simulink model "RT_TestMV_ATS"  (R2015b)
settings: Solver=FixedStepDiscrete  StartTime=0.0  StopTime=44.14  FixedStep=samplePeriod  RelTol=1e-3
PreLoadFcn:
  | initialize;
  | scramInitialize;
  | KR_alpha;
  | Discrete_Compensator;
  | ATS_setup
values from neighbouring files (symbols this model uses):
  a_ratio = K2/K1    (= 0.214196975539)    [KR_alpha.m]
  a_sub = ones(DOF_sub,1)    [KR_alpha.m]
  A_sub = (dt*alpha1_sub)/(Msub-Msub*alpha3_sub)    [KR_alpha.m]
  a_sup = ones(DOF_sup,1)    [KR_alpha.m]
  A_sup = (dt*alpha1_sup)/(Msup-Msup*alpha3_sup)    [KR_alpha.m]
  a_vector = ones(DOF,1)    [KR_alpha.m]
  alpha_f_sub = rho_inf_sub/(rho_inf_sub+1)    (= 0.5)    [KR_alpha.m]
  alpha_f_sup = rho_inf_sup/(rho_inf_sup+1)    (= 0.5)    [KR_alpha.m]
  B_sub = ((1/dt)*Msub*alpha3_sub)/alpha1_sub    [KR_alpha.m]
  B_sup = ((1/dt)*Msup*alpha3_sup)/alpha1_sup    [KR_alpha.m]
  controlPeriod = 1/2048    (= 0.00048828125)    [initialize.m]
  Csub = betaKinit*Ksub    [KR_alpha.m]
  Csup = (2*0.01/w1)*Ksup    (= 0.00743030767319)    [KR_alpha.m]
  D_sub = inv(alpha1_sub)/dt    [KR_alpha.m]
  D_sup = inv(alpha1_sup)/dt    [KR_alpha.m]
  dt = samplePeriod    [KR_alpha.m]
  forc_fbk_gain = 1.00    (= 1)    [KR_alpha.m]
  g = 386.089    [KR_alpha.m]
  gamma_sub = 0.5-alpha_m_sub+alpha_f_sub    (= 0.5)    [KR_alpha.m]
  gamma_sup = 0.5-alpha_m_sup+alpha_f_sup    (= 0.5)    [KR_alpha.m]
  K1 = 4.6686*K2    (= 9.3372)    [KR_alpha.m]
  K2 = 0.5*4    (= 2)    [KR_alpha.m]
  Ksub = Kstory    [KR_alpha.m]
  Msub = (0.88585/(56/450))*Mstory    (= 1.03248862309)    [KR_alpha.m]
  Msup = Mstory    (= 0.145044277356)    [KR_alpha.m]
  nAct = 4    [initialize.m]
  nDout = 4    [initialize.m]
  onesec = ceil(1/samplePeriod)    [Discrete_Compensator.m]
  samplePeriod = controlPeriod/upsampleFactor    (= 0.00048828125)    [initialize.m]
  scale_GM = 1.50    (= 1.5)    [KR_alpha.m]
  uy = 0.85    [KR_alpha.m]
undefined symbols (not defined in the file or in its folder): lhpNode, MRC, Nl, P_range, sample, SN, stsNode, Threshold, Zden, Znum
undefined symbols (not defined in the file): HybridCtrlParameters, Par
libraries: simulink x34, slrtlib x8, xpcsystranlib x5
(part 1 of 2)
CloseFcn:
  | rtwprivate ssgencode ModelCloseRequest scrnet_receiver
settings Model: SimulationMode=external  ExtModeArmWhenConnect=off  Creator=mvetsch  LastModifiedBy=Analyst-UCSD
settings SolverCC: EnableConcurrentExecution=on
settings DataIOCC: LimitDataPoints=off  SaveFormat=Array  SignalLoggingSaveFormat=ModelDataLogs  SignalLoggingName=sigsOut
settings OptimizationCC: BlockReduction=off  BooleanDataType=off  OptimizeBlockIOStorage=off  BufferReuse=off  GlobalBufferReuse=off  ExpressionFolding=off  ExpressionDepthLimit=2147483647  LocalBlockOutputs=off  InitFltsAndDblsToZero=on
settings DebuggingCC: SaveWithParameterizedLinksMsg=none  UnderspecifiedInitializationDetection=Classic  MergeDetectMultiDrivingBlocksExec=none  SignalResolutionControl=TryResolveAllWithWarning  MultiTaskDSMMsg=warning  MultiTaskCondExecSysMsg=none  FcnCallInpInsideContextMsg=UseLocalSettings  StateNameClashWarn=warning
settings HardwareCC: ProdBitPerPointer=32  ProdLargestAtomicFloat=None  ProdWordSize=32  ProdLongLongMode=on  ProdHWDeviceType=Generic->32-bit x86 compatible
settings RTWCC: SystemTargetFile=slrt.tlc  TemplateMakefile=slrt_default_tmf  Description=Simulink Real-Time  RTWCompilerOptimization=on
settings SimulinkRealTimeCC: TargetFcnLib=ansi_tfl_tmw.mat  RL32LogBufSizeModifier=10000000  RL32IRQSourceModifier=Auto (PCI only)  xPCIRQSourceBoard=Scramnet_SC150+
settings ConfigComp: CovModelRefEnable=Off

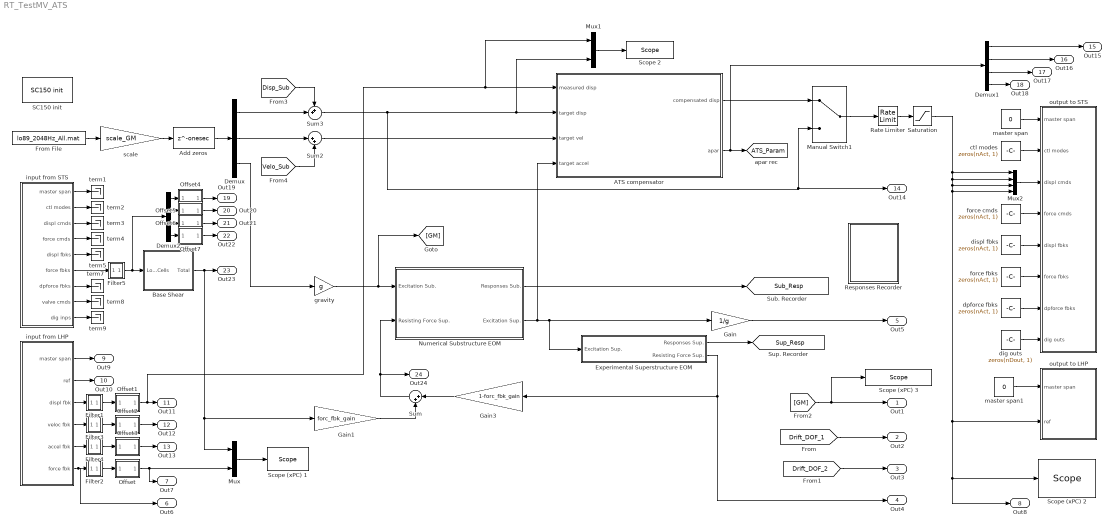
== system RT_TestMV_ATS ==
  ATS compensator : Subsystem  mask{param=Par}
      mask prompts: param "Initial a0, a1, a2 values :"
  Add zeros : Delay  DelayLength=onesec  InitialCondition=0
  Base Shear : Subsystem
  Demux : Demux  Outputs=3
  Demux1 : Demux
  Demux2 : Demux
  Experimental Superstructure EOM : Subsystem
  Filter1 : Subsystem
  Filter2 : Subsystem
  Filter3 : Subsystem
  Filter4 : Subsystem
  Filter5 : Subsystem
  From File : FromFile  FileName=lo89_2048Hz_All.mat  SampleTime=samplePeriod
  Gain : Gain  Gain=1/g
  Gain1 : Gain  Gain=forc_fbk_gain
  Gain3 : Gain  Gain=1-forc_fbk_gain
  Manual Switch1 : ManualSwitch
  Mux : Mux  Inputs=2
  Mux1 : Mux  Inputs=2
  Mux2 : Mux
  Numerical Substructure EOM : Subsystem
  Offset : Subsystem  mask(Signal Offset){nS=HybridCtrlParameters.nDOF, nOffset=onesec}
      mask prompts: nS "Number of Signals: nS"; nOffset "Number of samples to initialize offset: nOffset"
      mask help:
      | Offset signal by average of signal over initial number of samples.
      | Set nOffset = -1 for no signal offset.
      mask Display: fprintf('Signal\nOffset')
  Offset1 : Subsystem  mask(Signal Offset){nS=HybridCtrlParameters.nDOF, nOffset=onesec}
      mask prompts: nS "Number of Signals: nS"; nOffset "Number of samples to initialize offset: nOffset"
      mask help:
      | Offset signal by average of signal over initial number of samples.
      | Set nOffset = -1 for no signal offset.
      mask Display: fprintf('Signal\nOffset')
  Offset2 : Subsystem  mask(Signal Offset){nS=HybridCtrlParameters.nDOF, nOffset=onesec}
      mask prompts: nS "Number of Signals: nS"; nOffset "Number of samples to initialize offset: nOffset"
      mask help:
      | Offset signal by average of signal over initial number of samples.
      | Set nOffset = -1 for no signal offset.
      mask Display: fprintf('Signal\nOffset')
  Offset3 : Subsystem  mask(Signal Offset){nS=HybridCtrlParameters.nDOF, nOffset=onesec}
      mask prompts: nS "Number of Signals: nS"; nOffset "Number of samples to initialize offset: nOffset"
      mask help:
      | Offset signal by average of signal over initial number of samples.
      | Set nOffset = -1 for no signal offset.
      mask Display: fprintf('Signal\nOffset')
  Offset4 : Subsystem  mask(Signal Offset){nS=HybridCtrlParameters.nDOF, nOffset=onesec}
      mask prompts: nS "Number of Signals: nS"; nOffset "Number of samples to initialize offset: nOffset"
      mask help:
      | Offset signal by average of signal over initial number of samples.
      | Set nOffset = -1 for no signal offset.
      mask Display: fprintf('Signal\nOffset')
  Offset5 : Subsystem  mask(Signal Offset){nS=HybridCtrlParameters.nDOF, nOffset=onesec}
      mask prompts: nS "Number of Signals: nS"; nOffset "Number of samples to initialize offset: nOffset"
      mask help:
      | Offset signal by average of signal over initial number of samples.
      | Set nOffset = -1 for no signal offset.
      mask Display: fprintf('Signal\nOffset')
  Offset6 : Subsystem  mask(Signal Offset){nS=HybridCtrlParameters.nDOF, nOffset=onesec}
      mask prompts: nS "Number of Signals: nS"; nOffset "Number of samples to initialize offset: nOffset"
      mask help:
      | Offset signal by average of signal over initial number of samples.
      | Set nOffset = -1 for no signal offset.
      mask Display: fprintf('Signal\nOffset')
  Offset7 : Subsystem  mask(Signal Offset){nS=HybridCtrlParameters.nDOF, nOffset=onesec}
      mask prompts: nS "Number of Signals: nS"; nOffset "Number of samples to initialize offset: nOffset"
      mask help:
      | Offset signal by average of signal over initial number of samples.
      | Set nOffset = -1 for no signal offset.
      mask Display: fprintf('Signal\nOffset')
  Rate Limiter : RateLimiter  RisingSlewLimit=25  FallingSlewLimit=-25  SampleTimeMode=inherited
  Responses Recorder : Subsystem
  SC150 init : xpcsystranlib/Shared Memory/SC150 init   node=node  pci=-1
  Saturation : Saturate  UpperLimit=4.5  LowerLimit=-4.5
  Scope (xPC) 1 : slrtlib/Displays and Logging/Scope   scopeno=2  scopetype=Target  autostart=on  viewmode=Graphical redraw  formatstr='%15.6f'  grid=on  ylimits=[0,0]  nosamples=1024  noprepostsamples=0  interleave=1  triggermode=FreeRun  triggersignal=1  trigsignalfromport=off  triggerlevel=0.0  triggerslope=Either  triggerscope=1  triggersample=0  filename=data.dat  mode=Lazy  writesize=512  autorestart=off  dynamicfilemode=off  maxwritefilesize=512*1024^2
  Scope (xPC) 2 : slrtlib/Displays and Logging/Scope   scopeno=3  scopetype=Target  autostart=on  viewmode=Graphical redraw  formatstr='%15.6f'  grid=on  ylimits=[0,0]  nosamples=1024  noprepostsamples=0  interleave=1  triggermode=FreeRun  triggersignal=1  trigsignalfromport=off  triggerlevel=0.0  triggerslope=Either  triggerscope=1  triggersample=0  filename=data.dat  mode=Lazy  writesize=512  autorestart=off  dynamicfilemode=off  maxwritefilesize=512*1024^2
  Scope (xPC) 3 : slrtlib/Displays and Logging/Scope   scopeno=4  scopetype=Target  autostart=on  viewmode=Graphical redraw  formatstr='%15.6f'  grid=on  ylimits=[0,0]  nosamples=1024  noprepostsamples=0  interleave=1  triggermode=FreeRun  triggersignal=1  trigsignalfromport=off  triggerlevel=0.0  triggerslope=Either  triggerscope=1  triggersample=0  filename=data.dat  mode=Lazy  writesize=512  autorestart=off  dynamicfilemode=off  maxwritefilesize=512*1024^2
  Scope 2 : slrtlib/Displays and Logging/Scope   scopeno=1  scopetype=Target  autostart=on  viewmode=Graphical redraw  formatstr='%15.6f'  grid=on  ylimits=[0,0]  nosamples=250  noprepostsamples=0  interleave=1  triggermode=FreeRun  triggersignal=1  trigsignalfromport=off  triggerlevel=0.0  triggerslope=Either  triggerscope=1  triggersample=0  filename=data.dat  mode=Lazy  writesize=512  autorestart=off  dynamicfilemode=off  maxwritefilesize=512*1024^2
  Sum : Sum  Inputs=|++
  Sum2 : Sum  Inputs=|++
  Sum3 : Sum  Inputs=++|
  ctl modes : Constant  Value=zeros(nAct, 1)
  dig outs : Constant  Value=zeros(nDout, 1)  OutDataTypeStr=uint32
  displ fbks : Constant  Value=zeros(nAct, 1)
  dpforce fbks : Constant  Value=zeros(nAct, 1)
  force cmds : Constant  Value=zeros(nAct, 1)
  force fbks : Constant  Value=zeros(nAct, 1)
  gravity : Gain  Gain=g
  input from LHP : Subsystem
  input from STS : Subsystem
  master span : Constant  Value=0
  master span1 : Constant  Value=0
  output to LHP : Subsystem
  output to STS : Subsystem
  scale : Gain  Gain=scale_GM
  term{1..5,7..9} (8 alike) : Terminator
  Out1 : Outport  SampleTime=samplePeriod
  Out2 : Outport  Port=2  SampleTime=samplePeriod
  Out3 : Outport  Port=3  SampleTime=samplePeriod
  Out4 : Outport  Port=4  SampleTime=samplePeriod
  Out5 : Outport  Port=5  SampleTime=samplePeriod
  Out6 : Outport  Port=6  SampleTime=samplePeriod
  Out7 : Outport  Port=7  SampleTime=samplePeriod
  Out8 : Outport  Port=8  SampleTime=samplePeriod
  Out9 : Outport  Port=9  SampleTime=samplePeriod
  Out10 : Outport  Port=10  SampleTime=samplePeriod
  Out11 : Outport  Port=11  SampleTime=samplePeriod
  Out12 : Outport  Port=12  SampleTime=samplePeriod
  Out13 : Outport  Port=13  SampleTime=samplePeriod
  Out14 : Outport  Port=14
  Out15 : Outport  Port=15
  Out16 : Outport  Port=16
  Out17 : Outport  Port=17
  Out18 : Outport  Port=18
  Out19 : Outport  Port=19
  Out20 : Outport  Port=20
  Out21 : Outport  Port=21
  Out22 : Outport  Port=22
  Out23 : Outport  Port=23
  Out24 : Outport  Port=24
  tag scope: ATS_Param=global, Sub_Resp=global, Sup_Resp=global
  wires:
  master span/1 -> output to STS/1(master span)
  ctl modes/1 -> output to STS/2(ctl modes)
  force cmds/1 -> output to STS/4(force cmds)
  displ fbks/1 -> output to STS/5(displ fbks)
  force fbks/1 -> output to STS/6(force fbks)
  dpforce fbks/1 -> output to STS/7(dpforce fbks)
  input from STS/4(force cmds) -> term4/1
  input from STS/5(displ fbks) -> term5/1
  input from STS/6(force fbks) -> Filter5/1(In1)
  input from STS/7(dpforce fbks) -> term7/1
  input from STS/8(valve cmds) -> term8/1
  input from STS/9(dig inps) -> term9/1
  dig outs/1 -> output to STS/8(dig outs)
  input from LHP/1(master span) -> Out9/1
  input from LHP/3(displ fbk) -> Filter1/1(In1)
  input from LHP/4(veloc fbk) -> Filter3/1(In1)
  input from LHP/5(accel fbk) -> Filter4/1(In1)
  Mux/1 -> Scope (xPC) 1/1
  input from LHP/6(force fbk) -> Out6/1, Filter2/1(In1)
  Numerical Substructure EOM/1(Responses Sub.) -> [Sub_Resp]
  Experimental Superstructure EOM/1(Responses Sup.) -> [Sup_Resp]
  [Drift_DOF_1] -> Out2/1
  [Drift_DOF_2] -> Out3/1
  master span1/1 -> output to LHP/1(master span)
  Filter2/1(Out1) -> Offset/1(In1)
  Offset/1(Out1) -> Out7/1, Mux/2
  input from LHP/2(ref) -> Out10/1
  From File/1 -> scale/1
  gravity/1 -> [GM], Numerical Substructure EOM/1(Excitation Sub.)
  Sum/1 -> Out24/1, Numerical Substructure EOM/2(Resisting Force Sup.)
  Experimental Superstructure EOM/2(Resisting Force Sup.) -> Out4/1, Gain3/1
  [GM] -> Scope (xPC) 3/1, Out1/1
  Numerical Substructure EOM/2(Excitation Sup.) -> Gain/1, Experimental Superstructure EOM/1(Excitation Sup.), ATS compensator/4(target accel)
  Gain1/1 -> Sum/2
  Add zeros/1 -> Demux/1
  Demux/3 -> gravity/1
  [Disp_Sub] -> Sum3/1
  Gain/1 -> Out5/1
  scale/1 -> Add zeros/1
  input from STS/1(master span) -> term1/1
  Sum3/1 -> Mux1/2, ATS compensator/2(target disp), Manual Switch1/2, Out14/1
  Sum2/1 -> ATS compensator/3(target vel)
  Manual Switch1/1 -> Rate Limiter/1
  ATS compensator/1(compensated disp) -> Manual Switch1/1
  ATS compensator/2(apar) -> [ATS_Param], Demux1/1
  Rate Limiter/1 -> Saturation/1
  Saturation/1 -> Mux2/1, Mux2/2, Mux2/3, Mux2/4, Scope (xPC) 2/1, Out8/1, output to LHP/2(ref)
  Demux1/1 -> Out15/1
  Demux1/2 -> Out16/1
  Demux1/3 -> Out17/1
  Demux1/4 -> Out18/1
  Offset1/1(Out1) -> Mux1/1, ATS compensator/1(measured disp), Out11/1
  Gain3/1 -> Sum/1
  Filter1/1(Out1) -> Offset1/1(In1)
  Mux2/1 -> output to STS/3(displ cmds)
  input from STS/2(ctl modes) -> term2/1
  input from STS/3(displ cmds) -> term3/1
  Demux2/1 -> Offset4/1(In1)
  Demux2/2 -> Offset5/1(In1)
  Demux2/3 -> Offset6/1(In1)
  Demux2/4 -> Offset7/1(In1)
  Base Shear/1(Total) -> Mux/1, Gain1/1, Out23/1
  Filter3/1(Out1) -> Offset2/1(In1)
  Filter4/1(Out1) -> Offset3/1(In1)
  Offset2/1(Out1) -> Out12/1
  Offset3/1(Out1) -> Out13/1
  Filter5/1(Out1) -> Base Shear/1(Load Cells), Demux2/1
  Offset4/1(Out1) -> Out19/1
  Offset5/1(Out1) -> Out20/1
  Offset6/1(Out1) -> Out21/1
  Offset7/1(Out1) -> Out22/1
  Mux1/1 -> Scope 2/1
  Demux/2 -> Sum2/1
  [Velo_Sub] -> Sum2/2
  Demux/1 -> Sum3/2

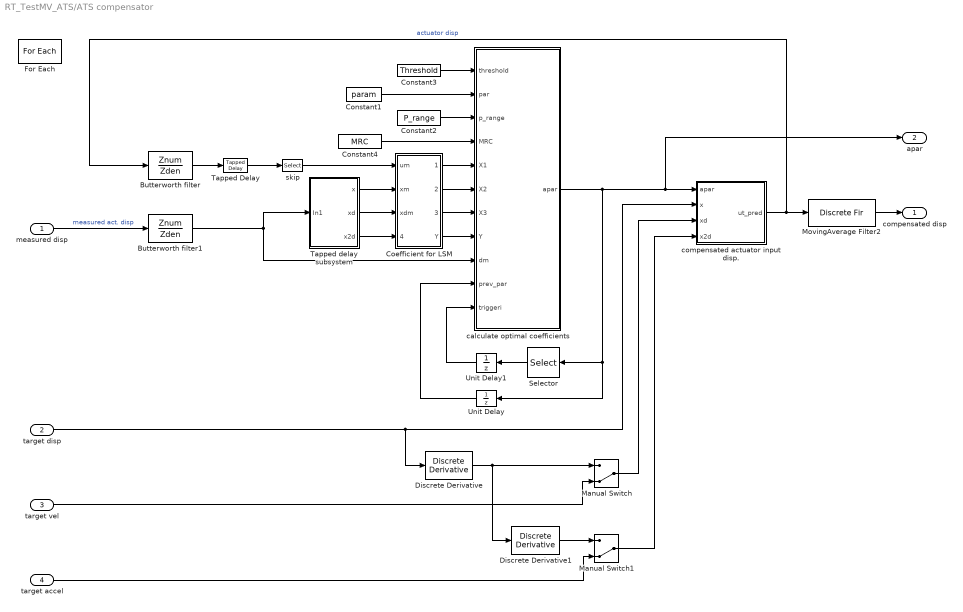
== system RT_TestMV_ATS/ATS compensator ==
  measured disp : Inport  Partition=on  PartitionDimension=1  PartitionWidth=1
  target disp : Inport  Port=2  Partition=on  PartitionDimension=1  PartitionWidth=1
  target vel : Inport  Port=3  Partition=on  PartitionDimension=1  PartitionWidth=1
  target accel : Inport  Port=4  Partition=on  PartitionDimension=1  PartitionWidth=1
  Butterworth filter : DiscreteTransferFcn  Numerator=Znum  Denominator=Zden  SampleTime=sample
  Butterworth filter1 : DiscreteTransferFcn  Numerator=Znum  Denominator=Zden  SampleTime=sample
  Coefficient for LSM : Subsystem
  Constant1 : Constant  Value=param
  Constant2 : Constant  Value=P_range
  Constant3 : Constant  Value=Threshold
  Constant4 : Constant  Value=MRC
  Discrete Derivative : simulink/Discrete/Discrete Derivative  gainval=1.0  ICPrevScaledInput=0.0  OutMin=[]  OutMax=[]  OutDataType=fixdt(1, 16)  OutScaling=2^-10  DoSatur=off
  Discrete Derivative1 : simulink/Discrete/Discrete Derivative  gainval=1.0  ICPrevScaledInput=0.0  OutMin=[]  OutMax=[]  OutDataType=fixdt(1, 16)  OutScaling=2^-10  DoSatur=off
  For Each : ForEach  DisableCoverage=on  IterateSubsysMaskParameter=on  SubsysMaskParameterIterationDimension=2  IndexMode=One-based
  Manual Switch : ManualSwitch  CurrentSetting=0
  Manual Switch1 : ManualSwitch  CurrentSetting=0
  MovingAverage Filter2 : DiscreteFir  Coefficients=1/numSample*ones(1,numSample)  mask(Moving Average Filter){numSample=10}
      mask prompts: numSample "Number of Samples: numSample"
      mask help:
      | Moving average filter by using discrete FIR filter.
      | Set numSample = 1 for no filtering.
      mask Display: fprintf('MovingAverage\nFilter')
  Selector : Selector  InputPortWidth=4  IndexOptions=Index vector (dialog)  Indices=4  OutputSizes=1
  Tapped Delay : simulink/Discrete/Tapped Delay  vinit=0.0  samptime=-1  NumDelays=Nl  DelayOrder=Oldest  includeCurrent=off
  Tapped delay subsystem : Subsystem
  Unit Delay : UnitDelay  SampleTime=-1
  Unit Delay1 : UnitDelay  SampleTime=-1
  calculate optimal coefficients : MATLAB Function  TreatAsAtomicUnit=on
  compensated actuator input disp. : MATLAB Function  TreatAsAtomicUnit=on
  skip : Selector  InputPortWidth=Nl  IndexOptions=Index vector (dialog)  Indices=[1:SN:Nl]  OutputSizes=1
  compensated disp : Outport  ConcatenationDimension=1
  apar : Outport  Port=2  ConcatenationDimension=1
  wires:
  measured disp/1 -> Butterworth filter1/1  "measured act. disp"
  Tapped Delay/1 -> skip/1
  calculate optimal coefficients/1(apar) -> Unit Delay/1, Selector/1, apar/1, compensated actuator input disp./1(apar)
  compensated actuator input disp./1(ut_pred) -> Butterworth filter/1, MovingAverage Filter2/1  "actuator disp"
  Constant1/1 -> calculate optimal coefficients/2(par)
  Constant2/1 -> calculate optimal coefficients/3(p_range)
  Unit Delay/1 -> calculate optimal coefficients/10(prev_par)
  target disp/1 -> compensated actuator input disp./2(x), Discrete Derivative/1
  skip/1 -> Coefficient for LSM/1(um)
  Tapped delay subsystem/1(x) -> Coefficient for LSM/2(xm)
  Tapped delay subsystem/2(xd) -> Coefficient for LSM/3(xdm)
  Tapped delay subsystem/3(x2d) -> Coefficient for LSM/4(x2dm)
  Coefficient for LSM/1(X(1,:)) -> calculate optimal coefficients/5(X1)
  Coefficient for LSM/2(X(2,:)) -> calculate optimal coefficients/6(X2)
  Coefficient for LSM/3(X(3,:)) -> calculate optimal coefficients/7(X3)
  Coefficient for LSM/4(Y) -> calculate optimal coefficients/8(Y)
  Unit Delay1/1 -> calculate optimal coefficients/11(triggeri)
  Constant3/1 -> calculate optimal coefficients/1(threshold)
  Butterworth filter/1 -> Tapped Delay/1
  Constant4/1 -> calculate optimal coefficients/4(MRC)
  Selector/1 -> Unit Delay1/1
  Manual Switch/1 -> compensated actuator input disp./3(xd)
  Discrete Derivative/1 -> Manual Switch/1, Discrete Derivative1/1
  target vel/1 -> Manual Switch/2
  Discrete Derivative1/1 -> Manual Switch1/1
  Manual Switch1/1 -> compensated actuator input disp./4(x2d)
  target accel/1 -> Manual Switch1/2
  Butterworth filter1/1 -> Tapped delay subsystem/1(In1), calculate optimal coefficients/9(dm)
  MovingAverage Filter2/1 -> compensated disp/1

== system RT_TestMV_ATS/Base Shear ==
  Load Cells : Inport
  Demux : Demux
  Offset1 : Subsystem  mask(Signal Offset){nS=HybridCtrlParameters.nDOF, nOffset=onesec}
      mask prompts: nS "Number of Signals: nS"; nOffset "Number of samples to initialize offset: nOffset"
      mask help:
      | Offset signal by average of signal over initial number of samples.
      | Set nOffset = -1 for no signal offset.
      mask Display: fprintf('Signal\nOffset')
  Offset2 : Subsystem  mask(Signal Offset){nS=HybridCtrlParameters.nDOF, nOffset=onesec}
      mask prompts: nS "Number of Signals: nS"; nOffset "Number of samples to initialize offset: nOffset"
      mask help:
      | Offset signal by average of signal over initial number of samples.
      | Set nOffset = -1 for no signal offset.
      mask Display: fprintf('Signal\nOffset')
  Offset3 : Subsystem  mask(Signal Offset){nS=HybridCtrlParameters.nDOF, nOffset=onesec}
      mask prompts: nS "Number of Signals: nS"; nOffset "Number of samples to initialize offset: nOffset"
      mask help:
      | Offset signal by average of signal over initial number of samples.
      | Set nOffset = -1 for no signal offset.
      mask Display: fprintf('Signal\nOffset')
  Offset4 : Subsystem  mask(Signal Offset){nS=HybridCtrlParameters.nDOF, nOffset=onesec}
      mask prompts: nS "Number of Signals: nS"; nOffset "Number of samples to initialize offset: nOffset"
      mask help:
      | Offset signal by average of signal over initial number of samples.
      | Set nOffset = -1 for no signal offset.
      mask Display: fprintf('Signal\nOffset')
  Sum : Sum  Inputs=++++
  Total : Outport
  wires:
  Demux/3 -> Offset2/1(In1)
  Demux/4 -> Offset3/1(In1)
  Demux/2 -> Offset1/1(In1)
  Demux/1 -> Offset4/1(In1)
  Load Cells/1 -> Demux/1
  Sum/1 -> Total/1
  Offset4/1(Out1) -> Sum/1
  Offset1/1(Out1) -> Sum/2
  Offset2/1(Out1) -> Sum/3
  Offset3/1(Out1) -> Sum/4

== system RT_TestMV_ATS/Experimental Superstructure EOM ==
  Excitation Sup. : Inport
  Delay1 : Delay  DelayLength=1
  Demux : Demux  Outputs=3
  Demux1 : Demux  Outputs=3
  Gain : Gain  Gain=Csup  Multiplication=Matrix(K*u) (u vector)
  Gain2 : Gain  Gain=-Msup*a_sup  Multiplication=Matrix(K*u)
  Material : Subsystem
  Subsystem : Subsystem
  Sum : Sum  Inputs=|++
  Terminator{,1..3} (4 alike) : Terminator
  Responses Sup. : Outport
  Resisting Force Sup. : Outport  Port=2
  wires:
  Subsystem/1(Responses i+1) -> Demux1/1, Demux/1, Delay1/1, Responses Sup./1
  Excitation Sup./1 -> Gain2/1
  Demux1/2 -> Gain/1
  Sum/1 -> Resisting Force Sup./1
  Demux/1 -> Material/1(Disp)
  Demux/3 -> Terminator/1
  Demux/2 -> Terminator1/1
  Demux1/1 -> Terminator2/1
  Demux1/3 -> Terminator3/1
  Gain/1 -> Sum/1
  Delay1/1 -> Subsystem/3(Responses i)
  Material/1(Force) -> Sum/2, Subsystem/2(Restoring A/E)
  Gain2/1 -> Subsystem/1(Excitation Force)

== system RT_TestMV_ATS/Filter1 ==
  In1 : Inport
  MovingAverage Filter2 : DiscreteFir  Coefficients=1/numSample*ones(1,numSample)  mask(Moving Average Filter){numSample=7}
      mask prompts: numSample "Number of Samples: numSample"
      mask help:
      | Moving average filter by using discrete FIR filter.
      | Set numSample = 1 for no filtering.
      mask Display: fprintf('MovingAverage\nFilter')
  Out1 : Outport
  wires:
  In1/1 -> MovingAverage Filter2/1
  MovingAverage Filter2/1 -> Out1/1

== system RT_TestMV_ATS/Filter2 ==
  In1 : Inport
  MovingAverage Filter2 : DiscreteFir  Coefficients=1/numSample*ones(1,numSample)  mask(Moving Average Filter){numSample=7}
      mask prompts: numSample "Number of Samples: numSample"
      mask help:
      | Moving average filter by using discrete FIR filter.
      | Set numSample = 1 for no filtering.
      mask Display: fprintf('MovingAverage\nFilter')
  Out1 : Outport
  wires:
  In1/1 -> MovingAverage Filter2/1
  MovingAverage Filter2/1 -> Out1/1

== system RT_TestMV_ATS/Filter3 ==
  In1 : Inport
  MovingAverage Filter2 : DiscreteFir  Coefficients=1/numSample*ones(1,numSample)  mask(Moving Average Filter){numSample=7}
      mask prompts: numSample "Number of Samples: numSample"
      mask help:
      | Moving average filter by using discrete FIR filter.
      | Set numSample = 1 for no filtering.
      mask Display: fprintf('MovingAverage\nFilter')
  Out1 : Outport
  wires:
  In1/1 -> MovingAverage Filter2/1
  MovingAverage Filter2/1 -> Out1/1

== system RT_TestMV_ATS/Filter4 ==
  In1 : Inport
  MovingAverage Filter2 : DiscreteFir  Coefficients=1/numSample*ones(1,numSample)  mask(Moving Average Filter){numSample=7}
      mask prompts: numSample "Number of Samples: numSample"
      mask help:
      | Moving average filter by using discrete FIR filter.
      | Set numSample = 1 for no filtering.
      mask Display: fprintf('MovingAverage\nFilter')
  Out1 : Outport
  wires:
  In1/1 -> MovingAverage Filter2/1
  MovingAverage Filter2/1 -> Out1/1

== system RT_TestMV_ATS/Filter5 ==
  In1 : Inport
  MovingAverage Filter2 : DiscreteFir  Coefficients=1/numSample*ones(1,numSample)  mask(Moving Average Filter){numSample=7}
      mask prompts: numSample "Number of Samples: numSample"
      mask help:
      | Moving average filter by using discrete FIR filter.
      | Set numSample = 1 for no filtering.
      mask Display: fprintf('MovingAverage\nFilter')
  Out1 : Outport
  wires:
  In1/1 -> MovingAverage Filter2/1
  MovingAverage Filter2/1 -> Out1/1

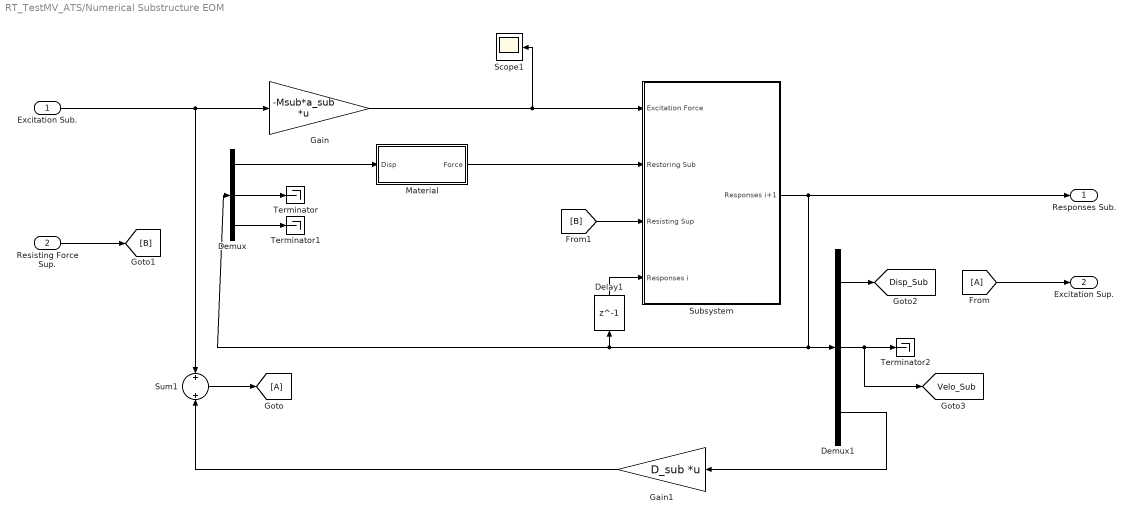
== system RT_TestMV_ATS/Numerical Substructure EOM ==
  Excitation Sub. : Inport
  Resisting Force Sup. : Inport  Port=2
  Delay1 : Delay  DelayLength=1
  Demux : Demux  Outputs=3
  Demux1 : Demux  Outputs=3
  Gain : Gain  Gain=-Msub*a_sub  Multiplication=Matrix(K*u)
  Gain1 : Gain  Gain=D_sub  Multiplication=Matrix(K*u) (u vector)
  Material : Subsystem
  Scope1 : Scope
  Subsystem : Subsystem
  Sum1 : Sum  Inputs=+||+
  Terminator : Terminator
  Terminator1 : Terminator
  Terminator2 : Terminator
  Responses Sub. : Outport
  Excitation Sup. : Outport  Port=2
  tag scope: Disp_Sub=global, Velo_Sub=global
  wires:
  Gain/1 -> Scope1/1, Subsystem/1(Excitation Force)
  Subsystem/1(Responses i+1) -> Demux/1, Delay1/1, Demux1/1, Responses Sub./1
  Demux/1 -> Material/1(Disp)
  Excitation Sub./1 -> Sum1/1, Gain/1
  Demux1/3 -> Gain1/1
  Demux/2 -> Terminator/1
  Demux/3 -> Terminator1/1
  Demux1/1 -> [Disp_Sub]
  Delay1/1 -> Subsystem/4(Responses i)
  Material/1(Force) -> Subsystem/2(Restoring Sub)
  Gain1/1 -> Sum1/2
  Demux1/2 -> [Velo_Sub], Terminator2/1
  Sum1/1 -> [A]
  [A] -> Excitation Sup./1
  Resisting Force Sup./1 -> [B]
  [B] -> Subsystem/3(Resisting Sup)

== system RT_TestMV_ATS/Offset ==
  In1 : Inport
  Constant : Constant  Value=zeros(1,nS)
  Counter : simulink/Sources/Counter Free-Running  NumBits=32  tsamp=-1
  Data Store Memory : DataStoreMemory  DataStoreName=x0  InitialValue=zeros(1,nS)  OutDataTypeStr=double
  Data Store Read : DataStoreRead  DataStoreName=x0  SampleTime=controlPeriod
  If : If  IfExpression=u1 < nOffset  ShowElse=off
  If Action : Subsystem  TreatAsAtomicUnit=on
  Sum1 : Sum  Inputs=+-|  SaturateOnIntegerOverflow=on  InputSameDT=on  OutDataTypeStr=Inherit: Same as first input
  Switch : Switch  Threshold=nOffset  SaturateOnIntegerOverflow=on  InputSameDT=on
  typeConv2 : DataTypeConversion  OutDataTypeStr=double  SaturateOnIntegerOverflow=on  RndMeth=Zero
  Out1 : Outport
  wires:
  Switch/1 -> Out1/1
  Sum1/1 -> Switch/1
  Data Store Read/1 -> Sum1/2
  In1/1 -> If Action/1(In1), Sum1/1
  Constant/1 -> Switch/3
  Counter/1 -> typeConv2/1
  If/1 -> If Action/Action
  typeConv2/1 -> Switch/2, If/1

== system RT_TestMV_ATS/Offset1 ==
  In1 : Inport
  Constant : Constant  Value=zeros(1,nS)
  Counter : simulink/Sources/Counter Free-Running  NumBits=32  tsamp=-1
  Data Store Memory : DataStoreMemory  DataStoreName=x0  InitialValue=zeros(1,nS)  OutDataTypeStr=double
  Data Store Read : DataStoreRead  DataStoreName=x0  SampleTime=controlPeriod
  If : If  IfExpression=u1 < nOffset  ShowElse=off
  If Action : Subsystem  TreatAsAtomicUnit=on
  Sum1 : Sum  Inputs=+-|  SaturateOnIntegerOverflow=on  InputSameDT=on  OutDataTypeStr=Inherit: Same as first input
  Switch : Switch  Threshold=nOffset  SaturateOnIntegerOverflow=on  InputSameDT=on
  typeConv2 : DataTypeConversion  OutDataTypeStr=double  SaturateOnIntegerOverflow=on  RndMeth=Zero
  Out1 : Outport
  wires:
  Switch/1 -> Out1/1
  Sum1/1 -> Switch/1
  Data Store Read/1 -> Sum1/2
  In1/1 -> If Action/1(In1), Sum1/1
  Constant/1 -> Switch/3
  Counter/1 -> typeConv2/1
  If/1 -> If Action/Action
  typeConv2/1 -> Switch/2, If/1

== system RT_TestMV_ATS/Offset2 ==
  In1 : Inport
  Constant : Constant  Value=zeros(1,nS)
  Counter : simulink/Sources/Counter Free-Running  NumBits=32  tsamp=-1
  Data Store Memory : DataStoreMemory  DataStoreName=x0  InitialValue=zeros(1,nS)  OutDataTypeStr=double
  Data Store Read : DataStoreRead  DataStoreName=x0  SampleTime=controlPeriod
  If : If  IfExpression=u1 < nOffset  ShowElse=off
  If Action : Subsystem  TreatAsAtomicUnit=on
  Sum1 : Sum  Inputs=+-|  SaturateOnIntegerOverflow=on  InputSameDT=on  OutDataTypeStr=Inherit: Same as first input
  Switch : Switch  Threshold=nOffset  SaturateOnIntegerOverflow=on  InputSameDT=on
  typeConv2 : DataTypeConversion  OutDataTypeStr=double  SaturateOnIntegerOverflow=on  RndMeth=Zero
  Out1 : Outport
  wires:
  Switch/1 -> Out1/1
  Sum1/1 -> Switch/1
  Data Store Read/1 -> Sum1/2
  In1/1 -> If Action/1(In1), Sum1/1
  Constant/1 -> Switch/3
  Counter/1 -> typeConv2/1
  If/1 -> If Action/Action
  typeConv2/1 -> Switch/2, If/1

== system RT_TestMV_ATS/Offset3 ==
  In1 : Inport
  Constant : Constant  Value=zeros(1,nS)
  Counter : simulink/Sources/Counter Free-Running  NumBits=32  tsamp=-1
  Data Store Memory : DataStoreMemory  DataStoreName=x0  InitialValue=zeros(1,nS)  OutDataTypeStr=double
  Data Store Read : DataStoreRead  DataStoreName=x0  SampleTime=controlPeriod
  If : If  IfExpression=u1 < nOffset  ShowElse=off
  If Action : Subsystem  TreatAsAtomicUnit=on
  Sum1 : Sum  Inputs=+-|  SaturateOnIntegerOverflow=on  InputSameDT=on  OutDataTypeStr=Inherit: Same as first input
  Switch : Switch  Threshold=nOffset  SaturateOnIntegerOverflow=on  InputSameDT=on
  typeConv2 : DataTypeConversion  OutDataTypeStr=double  SaturateOnIntegerOverflow=on  RndMeth=Zero
  Out1 : Outport
  wires:
  Switch/1 -> Out1/1
  Sum1/1 -> Switch/1
  Data Store Read/1 -> Sum1/2
  In1/1 -> If Action/1(In1), Sum1/1
  Constant/1 -> Switch/3
  Counter/1 -> typeConv2/1
  If/1 -> If Action/Action
  typeConv2/1 -> Switch/2, If/1

== system RT_TestMV_ATS/Offset4 ==
  In1 : Inport
  Constant : Constant  Value=zeros(1,nS)
  Counter : simulink/Sources/Counter Free-Running  NumBits=32  tsamp=-1
  Data Store Memory : DataStoreMemory  DataStoreName=x0  InitialValue=zeros(1,nS)  OutDataTypeStr=double
  Data Store Read : DataStoreRead  DataStoreName=x0  SampleTime=controlPeriod
  If : If  IfExpression=u1 < nOffset  ShowElse=off
  If Action : Subsystem  TreatAsAtomicUnit=on
  Sum1 : Sum  Inputs=+-|  SaturateOnIntegerOverflow=on  InputSameDT=on  OutDataTypeStr=Inherit: Same as first input
  Switch : Switch  Threshold=nOffset  SaturateOnIntegerOverflow=on  InputSameDT=on
  typeConv2 : DataTypeConversion  OutDataTypeStr=double  SaturateOnIntegerOverflow=on  RndMeth=Zero
  Out1 : Outport
  wires:
  Switch/1 -> Out1/1
  Sum1/1 -> Switch/1
  Data Store Read/1 -> Sum1/2
  In1/1 -> If Action/1(In1), Sum1/1
  Constant/1 -> Switch/3
  Counter/1 -> typeConv2/1
  If/1 -> If Action/Action
  typeConv2/1 -> Switch/2, If/1

== system RT_TestMV_ATS/Offset5 ==
  In1 : Inport
  Constant : Constant  Value=zeros(1,nS)
  Counter : simulink/Sources/Counter Free-Running  NumBits=32  tsamp=-1
  Data Store Memory : DataStoreMemory  DataStoreName=x0  InitialValue=zeros(1,nS)  OutDataTypeStr=double
  Data Store Read : DataStoreRead  DataStoreName=x0  SampleTime=controlPeriod
  If : If  IfExpression=u1 < nOffset  ShowElse=off
  If Action : Subsystem  TreatAsAtomicUnit=on
  Sum1 : Sum  Inputs=+-|  SaturateOnIntegerOverflow=on  InputSameDT=on  OutDataTypeStr=Inherit: Same as first input
  Switch : Switch  Threshold=nOffset  SaturateOnIntegerOverflow=on  InputSameDT=on
  typeConv2 : DataTypeConversion  OutDataTypeStr=double  SaturateOnIntegerOverflow=on  RndMeth=Zero
  Out1 : Outport
  wires:
  Switch/1 -> Out1/1
  Sum1/1 -> Switch/1
  Data Store Read/1 -> Sum1/2
  In1/1 -> If Action/1(In1), Sum1/1
  Constant/1 -> Switch/3
  Counter/1 -> typeConv2/1
  If/1 -> If Action/Action
  typeConv2/1 -> Switch/2, If/1

== system RT_TestMV_ATS/Offset6 ==
  In1 : Inport
  Constant : Constant  Value=zeros(1,nS)
  Counter : simulink/Sources/Counter Free-Running  NumBits=32  tsamp=-1
  Data Store Memory : DataStoreMemory  DataStoreName=x0  InitialValue=zeros(1,nS)  OutDataTypeStr=double
  Data Store Read : DataStoreRead  DataStoreName=x0  SampleTime=controlPeriod
  If : If  IfExpression=u1 < nOffset  ShowElse=off
  If Action : Subsystem  TreatAsAtomicUnit=on
  Sum1 : Sum  Inputs=+-|  SaturateOnIntegerOverflow=on  InputSameDT=on  OutDataTypeStr=Inherit: Same as first input
  Switch : Switch  Threshold=nOffset  SaturateOnIntegerOverflow=on  InputSameDT=on
  typeConv2 : DataTypeConversion  OutDataTypeStr=double  SaturateOnIntegerOverflow=on  RndMeth=Zero
  Out1 : Outport
  wires:
  Switch/1 -> Out1/1
  Sum1/1 -> Switch/1
  Data Store Read/1 -> Sum1/2
  In1/1 -> If Action/1(In1), Sum1/1
  Constant/1 -> Switch/3
  Counter/1 -> typeConv2/1
  If/1 -> If Action/Action
  typeConv2/1 -> Switch/2, If/1

== system RT_TestMV_ATS/Offset7 ==
  In1 : Inport
  Constant : Constant  Value=zeros(1,nS)
  Counter : simulink/Sources/Counter Free-Running  NumBits=32  tsamp=-1
  Data Store Memory : DataStoreMemory  DataStoreName=x0  InitialValue=zeros(1,nS)  OutDataTypeStr=double
  Data Store Read : DataStoreRead  DataStoreName=x0  SampleTime=controlPeriod
  If : If  IfExpression=u1 < nOffset  ShowElse=off
  If Action : Subsystem  TreatAsAtomicUnit=on
  Sum1 : Sum  Inputs=+-|  SaturateOnIntegerOverflow=on  InputSameDT=on  OutDataTypeStr=Inherit: Same as first input
  Switch : Switch  Threshold=nOffset  SaturateOnIntegerOverflow=on  InputSameDT=on
  typeConv2 : DataTypeConversion  OutDataTypeStr=double  SaturateOnIntegerOverflow=on  RndMeth=Zero
  Out1 : Outport
  wires:
  Switch/1 -> Out1/1
  Sum1/1 -> Switch/1
  Data Store Read/1 -> Sum1/2
  In1/1 -> If Action/1(In1), Sum1/1
  Constant/1 -> Switch/3
  Counter/1 -> typeConv2/1
  If/1 -> If Action/Action
  typeConv2/1 -> Switch/2, If/1

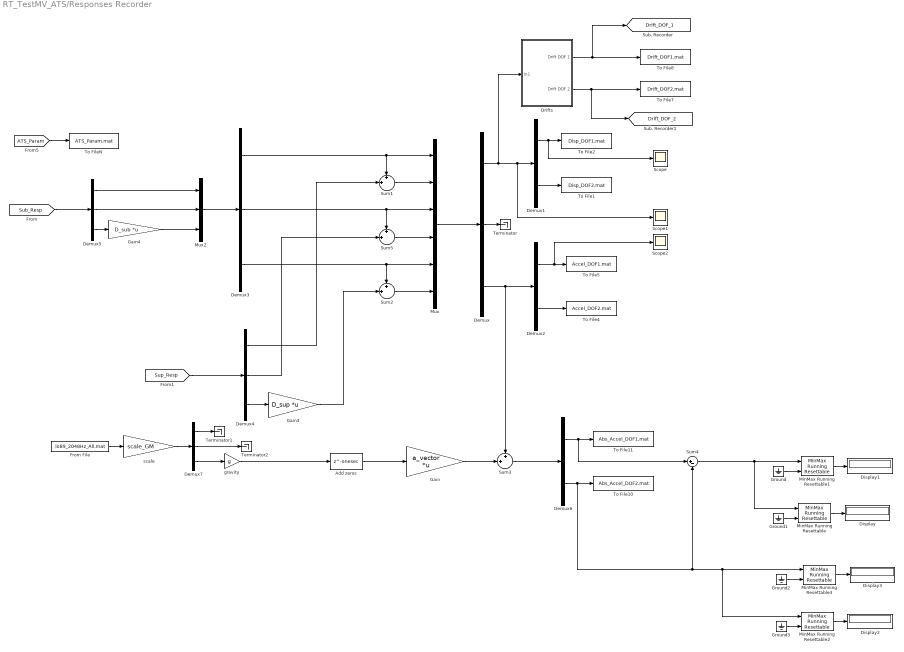
== system RT_TestMV_ATS/Responses Recorder ==
  Add zeros : Delay  DelayLength=onesec  InitialCondition=0
  Demux{,3..5,7} (5 alike) : Demux  Outputs=3
  Demux1 : Demux  Outputs=2
  Demux2 : Demux  Outputs=2
  Demux6 : Demux  Outputs=2
  Display{,1..3} (4 alike) : Display
  Drifts : Subsystem
  From File : FromFile  FileName=lo89_2048Hz_All.mat  SampleTime=samplePeriod
  Gain : Gain  Gain=a_vector  Multiplication=Matrix(K*u)
  Gain3 : Gain  Gain=D_sup  Multiplication=Matrix(K*u) (u vector)
  Gain4 : Gain  Gain=D_sub  Multiplication=Matrix(K*u) (u vector)
  Ground{,1..3} (4 alike) : Ground
  MinMax Running Resettable : simulink/Math Operations/MinMax Running Resettable  Function=max  vinit=0.0
  MinMax Running Resettable1 : simulink/Math Operations/MinMax Running Resettable  Function=min  vinit=0.0
  MinMax Running Resettable2 : simulink/Math Operations/MinMax Running Resettable  Function=max  vinit=0.0
  MinMax Running Resettable3 : simulink/Math Operations/MinMax Running Resettable  Function=min  vinit=0.0
  Mux : Mux  Inputs=6
  Mux2 : Mux  Inputs=3
  Scope : Scope
  Scope1 : Scope
  Scope2 : Scope
  Sum{1..3,5} (4 alike) : Sum  Inputs=+|+||
  Sum4 : Sum  Inputs=|+-
  Terminator : Terminator
  Terminator1 : Terminator
  Terminator2 : Terminator
  To File1 : ToFile  Filename=Disp_DOF2.mat
  To File10 : ToFile  Filename=Abs_Accel_DOF2.mat
  To File11 : ToFile  Filename=Abs_Accel_DOF1.mat
  To File2 : ToFile  Filename=Disp_DOF1.mat
  To File4 : ToFile  Filename=Accel_DOF2.mat
  To File5 : ToFile  Filename=Accel_DOF1.mat
  To File7 : ToFile  Filename=Drift_DOF2.mat  MatrixName=Drift_DOF2
  To File8 : ToFile  Filename=Drift_DOF1.mat  MatrixName=Drift_DOF1
  To FileN : ToFile  Filename=ATS_Param.mat  MatrixName=ats_param
  gravity : Gain  Gain=g
  scale : Gain  Gain=scale_GM
  tag scope: Drift_DOF_1=global, Drift_DOF_2=global
  wires:
  Demux1/2 -> To File1/1
  Demux2/1 -> Scope2/1, To File5/1
  Demux/3 -> Sum3/1, Demux2/1
  Demux1/1 -> Scope/1, To File2/1
  Demux/1 -> Drifts/1(In1), Scope1/1, Demux1/1
  [Sup_Resp] -> Demux4/1
  Mux/1 -> Demux/1
  Demux3/3 -> Sum2/1, Mux/5
  Demux4/3 -> Gain3/1
  Sum2/1 -> Mux/6
  Gain3/1 -> Sum2/2
  [Sub_Resp] -> Demux5/1
  Demux5/2 -> Mux2/2
  Demux5/1 -> Mux2/1
  Demux5/3 -> Gain4/1
  Gain4/1 -> Mux2/3
  Mux2/1 -> Demux3/1
  Demux/2 -> Terminator/1
  MinMax Running Resettable/1 -> Display/1
  MinMax Running Resettable1/1 -> Display1/1
  Ground/1 -> MinMax Running Resettable1/2
  Ground1/1 -> MinMax Running Resettable/2
  Demux2/2 -> To File4/1
  MinMax Running Resettable2/1 -> Display2/1
  MinMax Running Resettable3/1 -> Display3/1
  Ground2/1 -> MinMax Running Resettable3/2
  Ground3/1 -> MinMax Running Resettable2/2
  Drifts/1(Drift DOF 1) -> [Drift_DOF_1], To File8/1
  Drifts/2(Drift DOF 2) -> [Drift_DOF_2], To File7/1
  Gain/1 -> Sum3/2
  Sum3/1 -> Demux6/1
  gravity/1 -> Add zeros/1
  Demux3/1 -> Sum1/1, Mux/1
  Demux4/1 -> Sum1/2
  Sum1/1 -> Mux/2
  Demux3/2 -> Sum5/1, Mux/3
  Demux4/2 -> Sum5/2
  Sum5/1 -> Mux/4
  Demux6/1 -> Sum4/1, To File11/1
  Demux6/2 -> Sum4/2, MinMax Running Resettable2/1, MinMax Running Resettable3/1, To File10/1
  Sum4/1 -> MinMax Running Resettable/1, MinMax Running Resettable1/1
  Add zeros/1 -> Gain/1
  Demux7/3 -> gravity/1
  From File/1 -> scale/1
  Demux7/1 -> Terminator1/1
  Demux7/2 -> Terminator2/1
  [ATS_Param] -> To FileN/1
  scale/1 -> Demux7/1

== system RT_TestMV_ATS/input from LHP ==
  SC150 read : xpcsystranlib/Shared Memory/SC150 read   partition=lhpNode.Partitions(3:end)  errorport=off  ts=controlPeriod  pci=-1
  SC150 unpack : slrtlib/Shared Memory/Shared Memory Unpack   partition=lhpNode.Partitions(3:end)
  typeConv{1..6} (6 alike) : DataTypeConversion  OutDataTypeStr=double  SaturateOnIntegerOverflow=on  RndMeth=Zero
  master span : Outport
  ref : Outport  Port=2
  displ fbk : Outport  Port=3
  veloc fbk : Outport  Port=4
  accel fbk : Outport  Port=5
  force fbk : Outport  Port=6
  wires:
  SC150 unpack/6 -> typeConv6/1
  SC150 unpack/5 -> typeConv5/1
  SC150 unpack/4 -> typeConv4/1
  SC150 unpack/3 -> typeConv3/1
  SC150 unpack/2 -> typeConv2/1
  typeConv6/1 -> force fbk/1
  typeConv5/1 -> accel fbk/1
  typeConv4/1 -> veloc fbk/1
  typeConv3/1 -> displ fbk/1
  typeConv1/1 -> master span/1
  SC150 read/1 -> SC150 unpack/1
  typeConv2/1 -> ref/1
  SC150 unpack/1 -> typeConv1/1

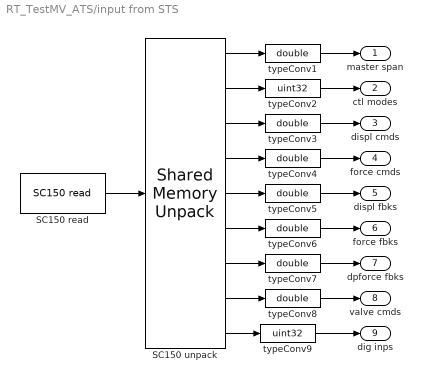
== system RT_TestMV_ATS/input from STS ==
  SC150 read : xpcsystranlib/Shared Memory/SC150 read   partition=stsNode.Partitions(9:end)  errorport=off  ts=controlPeriod  pci=-1
  SC150 unpack : slrtlib/Shared Memory/Shared Memory Unpack   partition=stsNode.Partitions(9:end)
  typeConv{1,3..8} (7 alike) : DataTypeConversion  OutDataTypeStr=double  SaturateOnIntegerOverflow=on  RndMeth=Zero
  typeConv2 : DataTypeConversion  OutDataTypeStr=uint32  SaturateOnIntegerOverflow=on  RndMeth=Zero
  typeConv9 : DataTypeConversion  OutDataTypeStr=uint32  SaturateOnIntegerOverflow=on  RndMeth=Zero
  master span : Outport
  ctl modes : Outport  Port=2
  displ cmds : Outport  Port=3
  force cmds : Outport  Port=4
  displ fbks : Outport  Port=5
  force fbks : Outport  Port=6
  dpforce fbks : Outport  Port=7
  valve cmds : Outport  Port=8
  dig inps : Outport  Port=9
  wires:
  SC150 unpack/8 -> typeConv8/1
  SC150 unpack/7 -> typeConv7/1
  SC150 unpack/6 -> typeConv6/1
  SC150 unpack/5 -> typeConv5/1
  SC150 unpack/4 -> typeConv4/1
  SC150 unpack/2 -> typeConv2/1
  typeConv2/1 -> ctl modes/1
  SC150 read/1 -> SC150 unpack/1
  typeConv1/1 -> master span/1
  typeConv3/1 -> displ cmds/1
  typeConv4/1 -> force cmds/1
  typeConv5/1 -> displ fbks/1
  typeConv6/1 -> force fbks/1
  typeConv7/1 -> dpforce fbks/1
  typeConv8/1 -> valve cmds/1
  SC150 unpack/9 -> typeConv9/1
  typeConv9/1 -> dig inps/1
  SC150 unpack/3 -> typeConv3/1
  SC150 unpack/1 -> typeConv1/1

== system RT_TestMV_ATS/output to LHP ==
  master span : Inport
  ref : Inport  Port=2
  SC150 pack : slrtlib/Shared Memory/Shared Memory Pack   partition=lhpNode.Partitions(1:2)
  SC150 write : xpcsystranlib/Shared Memory/SC150 write   partition=lhpNode.Partitions(1:2)  errorport=off  ts=controlPeriod  pci=-1
  typeConv1 : DataTypeConversion  OutDataTypeStr=single  SaturateOnIntegerOverflow=on  RndMeth=Zero
  typeConv2 : DataTypeConversion  OutDataTypeStr=single  SaturateOnIntegerOverflow=on  RndMeth=Zero
  wires:
  master span/1 -> typeConv1/1
  SC150 pack/1 -> SC150 write/1
  ref/1 -> typeConv2/1
  typeConv1/1 -> SC150 pack/1
  typeConv2/1 -> SC150 pack/2

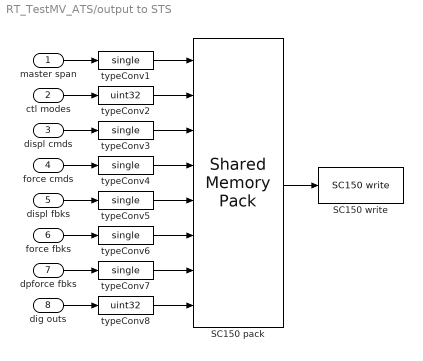
== system RT_TestMV_ATS/output to STS ==
  master span : Inport
  ctl modes : Inport  Port=2
  displ cmds : Inport  Port=3
  force cmds : Inport  Port=4
  displ fbks : Inport  Port=5
  force fbks : Inport  Port=6
  dpforce fbks : Inport  Port=7
  dig outs : Inport  Port=8
  SC150 pack : slrtlib/Shared Memory/Shared Memory Pack   partition=stsNode.Partitions(1:8)
  SC150 write : xpcsystranlib/Shared Memory/SC150 write   partition=stsNode.Partitions(1:8)  errorport=off  ts=controlPeriod  pci=-1
  typeConv{1,3..7} (6 alike) : DataTypeConversion  OutDataTypeStr=single  SaturateOnIntegerOverflow=on  RndMeth=Zero
  typeConv2 : DataTypeConversion  OutDataTypeStr=uint32  SaturateOnIntegerOverflow=on  RndMeth=Zero
  typeConv8 : DataTypeConversion  OutDataTypeStr=uint32  SaturateOnIntegerOverflow=on  RndMeth=Zero
  wires:
  typeConv4/1 -> SC150 pack/4
  typeConv3/1 -> SC150 pack/3
  typeConv2/1 -> SC150 pack/2
  typeConv1/1 -> SC150 pack/1
  ctl modes/1 -> typeConv2/1
  displ cmds/1 -> typeConv3/1
  SC150 pack/1 -> SC150 write/1
  master span/1 -> typeConv1/1
  force cmds/1 -> typeConv4/1
  displ fbks/1 -> typeConv5/1
  force fbks/1 -> typeConv6/1
  dpforce fbks/1 -> typeConv7/1
  typeConv5/1 -> SC150 pack/5
  typeConv6/1 -> SC150 pack/6
  typeConv7/1 -> SC150 pack/7
  typeConv8/1 -> SC150 pack/8
  dig outs/1 -> typeConv8/1

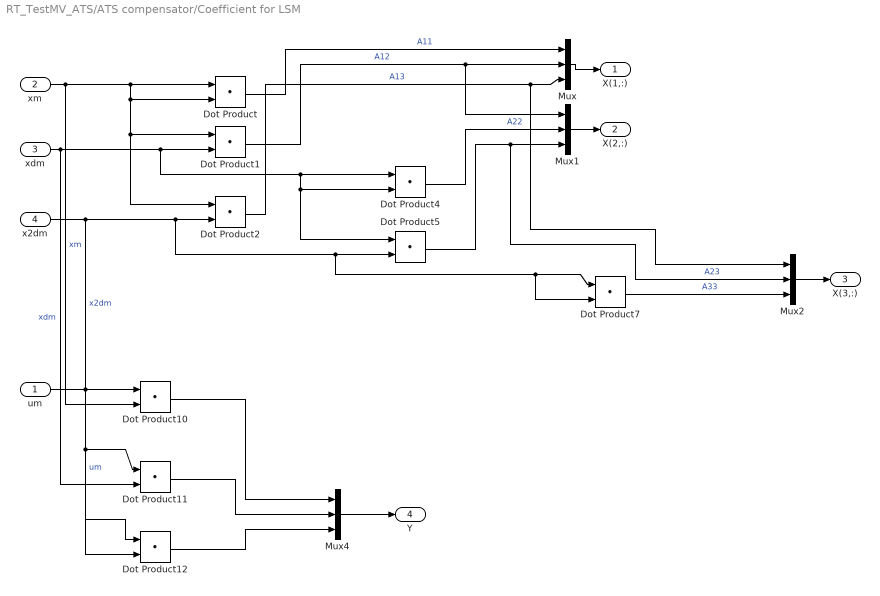
== system RT_TestMV_ATS/ATS compensator/Coefficient for LSM ==
  um : Inport
  xm : Inport  Port=2
  xdm : Inport  Port=3
  x2dm : Inport  Port=4
  Dot Product{,1..2,4..5,7,10..12} (9 alike) : DotProduct  InputSameDT=on  OutDataTypeStr=Inherit: Inherit via internal rule
  Mux{,1..2,4} (4 alike) : Mux  Inputs=3
  X(1,:) : Outport
  X(2,:) : Outport  Port=2
  X(3,:) : Outport  Port=3
  Y : Outport  Port=4
  wires:
  xm/1 -> Dot Product/1, Dot Product/2, Dot Product1/1, Dot Product2/1, Dot Product10/2  "xm"
  xdm/1 -> Dot Product1/2, Dot Product4/1, Dot Product4/2, Dot Product5/1, Dot Product11/2  "xdm"
  x2dm/1 -> Dot Product2/2, Dot Product5/2, Dot Product7/1, Dot Product7/2, Dot Product12/2  "x2dm"
  um/1 -> Dot Product10/1, Dot Product11/1, Dot Product12/1  "um"
  Dot Product/1 -> Mux/1  "A11"
  Dot Product1/1 -> Mux/2, Mux1/1  "A12"
  Dot Product2/1 -> Mux/3, Mux2/1  "A13"
  Mux/1 -> X(1,:)/1
  Dot Product4/1 -> Mux1/2  "A22"
  Dot Product5/1 -> Mux1/3, Mux2/2  "A23"
  Mux1/1 -> X(2,:)/1
  Dot Product7/1 -> Mux2/3  "A33"
  Mux2/1 -> X(3,:)/1
  Mux4/1 -> Y/1
  Dot Product10/1 -> Mux4/1
  Dot Product11/1 -> Mux4/2
  Dot Product12/1 -> Mux4/3

== system RT_TestMV_ATS/ATS compensator/Tapped delay subsystem ==
  In1 : Inport
  Discrete Derivative : simulink/Discrete/Discrete Derivative  gainval=1.0  ICPrevScaledInput=0.0  OutMin=[]  OutMax=[]  OutDataType=fixdt(1, 16)  OutScaling=2^-10  DoSatur=off
  Discrete Derivative1 : simulink/Discrete/Discrete Derivative  gainval=1.0  ICPrevScaledInput=0.0  OutMin=[]  OutMax=[]  OutDataType=fixdt(1, 16)  OutScaling=2^-10  DoSatur=off
  Tapped Delay : simulink/Discrete/Tapped Delay  vinit=0.0  samptime=-1  NumDelays=Nl  DelayOrder=Oldest  includeCurrent=off
  Tapped Delay1 : simulink/Discrete/Tapped Delay  vinit=0.0  samptime=-1  NumDelays=Nl  DelayOrder=Oldest  includeCurrent=off
  Tapped Delay2 : simulink/Discrete/Tapped Delay  vinit=0.0  samptime=-1  NumDelays=Nl  DelayOrder=Oldest  includeCurrent=off
  skip : Selector  InputPortWidth=Nl  IndexOptions=Index vector (dialog)  Indices=[1:SN:Nl]  OutputSizes=1
  skip1 : Selector  InputPortWidth=Nl  IndexOptions=Index vector (dialog)  Indices=[1:SN:Nl]  OutputSizes=1
  skip2 : Selector  InputPortWidth=Nl  IndexOptions=Index vector (dialog)  Indices=[1:SN:Nl]  OutputSizes=1
  x : Outport
  xd : Outport  Port=2
  x2d : Outport  Port=3
  wires:
  In1/1 -> Discrete Derivative/1, Tapped Delay/1
  Discrete Derivative/1 -> Discrete Derivative1/1, Tapped Delay1/1
  Discrete Derivative1/1 -> Tapped Delay2/1
  Tapped Delay/1 -> skip/1
  Tapped Delay1/1 -> skip1/1
  Tapped Delay2/1 -> skip2/1
  skip/1 -> x/1
  skip1/1 -> xd/1
  skip2/1 -> x2d/1

== system RT_TestMV_ATS/Base Shear/Offset1 ==
  In1 : Inport
  Constant : Constant  Value=zeros(1,nS)
  Counter : simulink/Sources/Counter Free-Running  NumBits=32  tsamp=-1
  Data Store Memory : DataStoreMemory  DataStoreName=x0  InitialValue=zeros(1,nS)  OutDataTypeStr=double
  Data Store Read : DataStoreRead  DataStoreName=x0  SampleTime=controlPeriod
  If : If  IfExpression=u1 < nOffset  ShowElse=off
  If Action : Subsystem  TreatAsAtomicUnit=on
  Sum1 : Sum  Inputs=+-|  SaturateOnIntegerOverflow=on  InputSameDT=on  OutDataTypeStr=Inherit: Same as first input
  Switch : Switch  Threshold=nOffset  SaturateOnIntegerOverflow=on  InputSameDT=on
  typeConv2 : DataTypeConversion  OutDataTypeStr=double  SaturateOnIntegerOverflow=on  RndMeth=Zero
  Out1 : Outport
  wires:
  Switch/1 -> Out1/1
  Sum1/1 -> Switch/1
  Data Store Read/1 -> Sum1/2
  In1/1 -> If Action/1(In1), Sum1/1
  Constant/1 -> Switch/3
  Counter/1 -> typeConv2/1
  If/1 -> If Action/Action
  typeConv2/1 -> Switch/2, If/1

== system RT_TestMV_ATS/Base Shear/Offset2 ==
  In1 : Inport
  Constant : Constant  Value=zeros(1,nS)
  Counter : simulink/Sources/Counter Free-Running  NumBits=32  tsamp=-1
  Data Store Memory : DataStoreMemory  DataStoreName=x0  InitialValue=zeros(1,nS)  OutDataTypeStr=double
  Data Store Read : DataStoreRead  DataStoreName=x0  SampleTime=controlPeriod
  If : If  IfExpression=u1 < nOffset  ShowElse=off
  If Action : Subsystem  TreatAsAtomicUnit=on
  Sum1 : Sum  Inputs=+-|  SaturateOnIntegerOverflow=on  InputSameDT=on  OutDataTypeStr=Inherit: Same as first input
  Switch : Switch  Threshold=nOffset  SaturateOnIntegerOverflow=on  InputSameDT=on
  typeConv2 : DataTypeConversion  OutDataTypeStr=double  SaturateOnIntegerOverflow=on  RndMeth=Zero
  Out1 : Outport
  wires:
  Switch/1 -> Out1/1
  Sum1/1 -> Switch/1
  Data Store Read/1 -> Sum1/2
  In1/1 -> If Action/1(In1), Sum1/1
  Constant/1 -> Switch/3
  Counter/1 -> typeConv2/1
  If/1 -> If Action/Action
  typeConv2/1 -> Switch/2, If/1

== system RT_TestMV_ATS/Base Shear/Offset3 ==
  In1 : Inport
  Constant : Constant  Value=zeros(1,nS)
  Counter : simulink/Sources/Counter Free-Running  NumBits=32  tsamp=-1
  Data Store Memory : DataStoreMemory  DataStoreName=x0  InitialValue=zeros(1,nS)  OutDataTypeStr=double
  Data Store Read : DataStoreRead  DataStoreName=x0  SampleTime=controlPeriod
  If : If  IfExpression=u1 < nOffset  ShowElse=off
  If Action : Subsystem  TreatAsAtomicUnit=on
  Sum1 : Sum  Inputs=+-|  SaturateOnIntegerOverflow=on  InputSameDT=on  OutDataTypeStr=Inherit: Same as first input
  Switch : Switch  Threshold=nOffset  SaturateOnIntegerOverflow=on  InputSameDT=on
  typeConv2 : DataTypeConversion  OutDataTypeStr=double  SaturateOnIntegerOverflow=on  RndMeth=Zero
  Out1 : Outport
  wires:
  Switch/1 -> Out1/1
  Sum1/1 -> Switch/1
  Data Store Read/1 -> Sum1/2
  In1/1 -> If Action/1(In1), Sum1/1
  Constant/1 -> Switch/3
  Counter/1 -> typeConv2/1
  If/1 -> If Action/Action
  typeConv2/1 -> Switch/2, If/1

== system RT_TestMV_ATS/Base Shear/Offset4 ==
  In1 : Inport
  Constant : Constant  Value=zeros(1,nS)
  Counter : simulink/Sources/Counter Free-Running  NumBits=32  tsamp=-1
  Data Store Memory : DataStoreMemory  DataStoreName=x0  InitialValue=zeros(1,nS)  OutDataTypeStr=double
  Data Store Read : DataStoreRead  DataStoreName=x0  SampleTime=controlPeriod
  If : If  IfExpression=u1 < nOffset  ShowElse=off
  If Action : Subsystem  TreatAsAtomicUnit=on
  Sum1 : Sum  Inputs=+-|  SaturateOnIntegerOverflow=on  InputSameDT=on  OutDataTypeStr=Inherit: Same as first input
  Switch : Switch  Threshold=nOffset  SaturateOnIntegerOverflow=on  InputSameDT=on
  typeConv2 : DataTypeConversion  OutDataTypeStr=double  SaturateOnIntegerOverflow=on  RndMeth=Zero
  Out1 : Outport
  wires:
  Switch/1 -> Out1/1
  Sum1/1 -> Switch/1
  Data Store Read/1 -> Sum1/2
  In1/1 -> If Action/1(In1), Sum1/1
  Constant/1 -> Switch/3
  Counter/1 -> typeConv2/1
  If/1 -> If Action/Action
  typeConv2/1 -> Switch/2, If/1

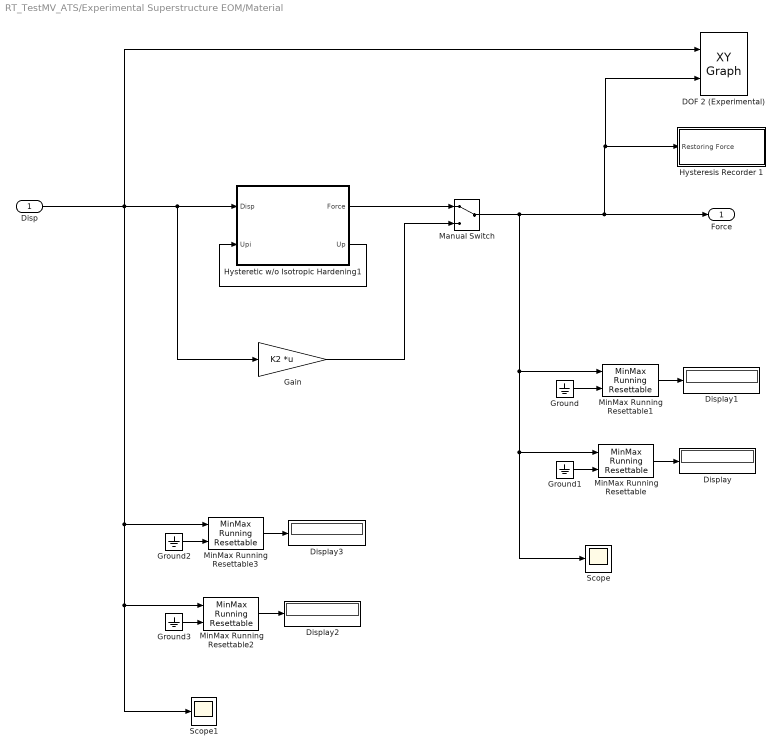
== system RT_TestMV_ATS/Experimental Superstructure EOM/Material ==
  Disp : Inport
  DOF 2 (Experimental) : simulink/Sinks/XY Graph  xmin=-6  xmax=6  ymin=-25  ymax=25  st=-1
  Display{,1..3} (4 alike) : Display
  Gain : Gain  Gain=K2  Multiplication=Matrix(K*u) (u vector)
  Ground{,1..3} (4 alike) : Ground
  Hysteresis Recorder 1 : Subsystem
  Hysteretic w/o Isotropic Hardening1 : Subsystem
  Manual Switch : ManualSwitch
  MinMax Running Resettable : simulink/Math Operations/MinMax Running Resettable  Function=max  vinit=0.0
  MinMax Running Resettable1 : simulink/Math Operations/MinMax Running Resettable  Function=min  vinit=0.0
  MinMax Running Resettable2 : simulink/Math Operations/MinMax Running Resettable  Function=max  vinit=0.0
  MinMax Running Resettable3 : simulink/Math Operations/MinMax Running Resettable  Function=min  vinit=0.0
  Scope : Scope
  Scope1 : Scope
  Force : Outport
  wires:
  Hysteretic w/o Isotropic Hardening1/2(Up) -> Hysteretic w/o Isotropic Hardening1/2(Upi)
  Hysteretic w/o Isotropic Hardening1/1(Force) -> Manual Switch/1
  Gain/1 -> Manual Switch/2
  MinMax Running Resettable2/1 -> Display2/1
  Ground/1 -> MinMax Running Resettable1/2
  Ground2/1 -> MinMax Running Resettable3/2
  Ground1/1 -> MinMax Running Resettable/2
  MinMax Running Resettable1/1 -> Display1/1
  MinMax Running Resettable/1 -> Display/1
  Ground3/1 -> MinMax Running Resettable2/2
  Manual Switch/1 -> MinMax Running Resettable1/1, MinMax Running Resettable/1, Scope/1, DOF 2 (Experimental)/2, Hysteresis Recorder 1/1(Restoring Force), Force/1
  MinMax Running Resettable3/1 -> Display3/1
  Disp/1 -> DOF 2 (Experimental)/1, MinMax Running Resettable3/1, MinMax Running Resettable2/1, Scope1/1, Gain/1, Hysteretic w/o Isotropic Hardening1/1(Disp)

== system RT_TestMV_ATS/Experimental Superstructure EOM/Subsystem ==
  Excitation Force : Inport
  Restoring A/E : Inport  Port=2
  Responses i : Inport  Port=3
  Delay : Delay  DelayLength=1
  Delay1 : Delay  DelayLength=1
  Gain : Gain  Gain=1-alpha_f_sup
  Gain1 : Gain  Gain=alpha_f_sup
  Gain2 : Gain  Gain=1-alpha_f_sup
  Gain3 : Gain  Gain=alpha_f_sup
  Mux : Mux  Inputs=3
  Subsystem : Subsystem
  Subsystem1 : Subsystem
  Subsystem2 : Subsystem
  Sum : Sum
  Sum1 : Sum
  Responses i+1 : Outport
  wires:
  Excitation Force/1 -> Delay/1, Gain/1
  Delay/1 -> Gain1/1
  Gain/1 -> Sum/1
  Gain1/1 -> Sum/2
  Sum/1 -> Subsystem2/2(F i+1-alpha_f)
  Mux/1 -> Responses i+1/1
  Subsystem1/1(X' i+1) -> Mux/2
  Subsystem/1(X i+1) -> Mux/1
  Subsystem2/1(X'hat i+1) -> Mux/3
  Delay1/1 -> Gain3/1
  Gain2/1 -> Sum1/1
  Gain3/1 -> Sum1/2
  Sum1/1 -> Subsystem2/3(R i+1-alpha_f)
  Responses i/1 -> Subsystem2/1(In), Subsystem1/1(In), Subsystem/1(In)
  Restoring A/E/1 -> Delay1/1, Gain2/1
